simulink model "IEEE34_PMSG"  (R2024a)
settings: Solver=FixedStepDiscrete  StartTime=0.0  StopTime=ttotal  RelTol=1e-3
values from neighbouring files (symbols this model uses):
  C0_300 = 4.9597e-09    [Data_input_DFIG.mat]    (also in Data_input_PMSG.mat)
  C0_301 = 4.8339e-09    [Data_input_DFIG.mat]    (also in Data_input_PMSG.mat)
  C1_300 = 1.0146e-08    [Data_input_DFIG.mat]    (also in Data_input_PMSG.mat)
  C1_301 = 9.7319e-09    [Data_input_DFIG.mat]    (also in Data_input_PMSG.mat)
  CC = [20000 9000 135000 20000 150000 10000 16000 7000 105000 16000 75000 5000 ... (36 elements, 6x6)]    [Data_input_DFIG.mat]    (also in Data_input_PMSG.mat)
  CD = [0 0 34000 135000 0 0 0 7000 0 7000 2000 4000 ... (114 elements, 19x6)]    [Data_input_DFIG.mat]    (also in Data_input_PMSG.mat)
  cte = 1e-06    [Data_input_DFIG.mat]    (also in Data_input_PMSG.mat)
  L0_300 = 0.0039    [Data_input_DFIG.mat]    (also in Data_input_PMSG.mat)
  L0_301 = 0.0043    [Data_input_DFIG.mat]    (also in Data_input_PMSG.mat)
  L1_300 = 0.0014    [Data_input_DFIG.mat]    (also in Data_input_PMSG.mat)
  L1_301 = 0.0014    [Data_input_DFIG.mat]    (also in Data_input_PMSG.mat)
  R0_300 = 1.0909    [Data_input_DFIG.mat]    (also in Data_input_PMSG.mat)
  R0_301 = 1.4885    [Data_input_DFIG.mat]    (also in Data_input_PMSG.mat)
  R1_300 = 0.6983    [Data_input_DFIG.mat]    (also in Data_input_PMSG.mat)
  R1_301 = 1.0537    [Data_input_DFIG.mat]    (also in Data_input_PMSG.mat)
  tf_AB = 1.75    [Data_input_DFIG.mat]    (also in Data_input_PMSG.mat = 2.65)
  tf_ABC = 1.75    [Data_input_DFIG.mat]    (also in Data_input_PMSG.mat = 2.65)
  tf_ABT = 1.75    [Data_input_DFIG.mat]    (also in Data_input_PMSG.mat = 2.65)
  tf_AT = 1.75    [Data_input_DFIG.mat]    (also in Data_input_PMSG.mat = 2.65)
  tf_BC = 1.75    [Data_input_DFIG.mat]    (also in Data_input_PMSG.mat = 2.65)
  tf_BCT = 1.75    [Data_input_DFIG.mat]    (also in Data_input_PMSG.mat = 2.65)
  tf_BT = 1.75    [Data_input_DFIG.mat]    (also in Data_input_PMSG.mat = 2.65)
  tf_CA = 1.75    [Data_input_DFIG.mat]    (also in Data_input_PMSG.mat = 2.65)
  tf_CAT = 1.75    [Data_input_DFIG.mat]    (also in Data_input_PMSG.mat = 2.65)
  tf_CT = 1.75    [Data_input_DFIG.mat]    (also in Data_input_PMSG.mat = 2.65)
  Ts = 5.008e-06    [Data_input_DFIG.mat]    (also in Data_input_PMSG.mat = 1.0016e-05)
undefined symbols (not defined in the file or in its folder): D1, Delta, DiscIntNeverNeededParam, find_system
libraries: spsThreePhaseSeriesRLCLoadLib x31, spsThreePhasePISectionLineLib x22, spsGroundLib x15, spsSeriesRLCLoadLib x14, spsThreePhaseFaultLib x10, spsSecondOrderFilterLib x9, spsPiSectionLineLib x8, spsThreePhaseVIMeasurementLib x6, spsabctodq0Lib x5, simulink_extras x4, spsFirstOrderFilterLib x4, spsThreePhaseTransformerTwoWindingsLib x3
(part 4 of 4)

== system IEEE34_PMSG/Wind Turbine Type 4/Control/Measurement and Transformation/Discrete 3-phase PLL-Driven Positive-Sequence Active & Reactive Power/Discrete 3-phase PLL-Driven Positive-Sequence Fundamental Value/Discrete Variable Frequency Mean value2/Correction subsystem ==
  N : Inport
  F : Inport  Port=2
  In : Inport  Port=3
  Gain1 : Gain  Gain=0.5  SaturateOnIntegerOverflow=on  OutDataTypeStr=Inherit: Same as input  ParamDataTypeStr=Inherit: Same as input
  Product2 : Product  Inputs=*/  InputSameDT=on  SaturateOnIntegerOverflow=on  OutDataTypeStr=Inherit: Same as first input
  Product4 : Product  Inputs=**  InputSameDT=on  SaturateOnIntegerOverflow=on  OutDataTypeStr=Inherit: Same as first input
  Product5 : Product  Inputs=**  InputSameDT=on  SaturateOnIntegerOverflow=on  OutDataTypeStr=Inherit: Same as first input
  Sum1 : Sum  Inputs=+-  InputSameDT=on  SaturateOnIntegerOverflow=on  OutDataTypeStr=Inherit: Same as first input
  Sum4 : Sum  InputSameDT=on  SaturateOnIntegerOverflow=on  OutDataTypeStr=Inherit: Same as first input
  Sum5 : Sum  Inputs=+-  InputSameDT=on  SaturateOnIntegerOverflow=on  OutDataTypeStr=Inherit: Same as first input
  Unit Delay : UnitDelay  SampleTime=Ts  HasFrameUpgradeWarning=on
  Out : Outport  VectorParamsAs1DForOutWhenUnconnected=off
  wires:
  Product4/1 -> Out/1
  Sum4/1 -> Product4/2
  Gain1/1 -> Sum4/1
  Product5/1 -> Gain1/1
  Sum1/1 -> Product5/2
  In/1 -> Sum4/2, Unit Delay/1, Sum1/1
  Product2/1 -> Product4/1
  Sum5/1 -> Product5/1, Product2/1
  F/1 -> Sum5/2
  N/1 -> Product2/2, Sum5/1
  Unit Delay/1 -> Sum1/2

== system IEEE34_PMSG/Wind Turbine Type 4/Control/Measurement and Transformation/Discrete 3-phase PLL-Driven Positive-Sequence Active & Reactive Power/Discrete 3-phase PLL-Driven Positive-Sequence Fundamental Value/Discrete Variable Frequency Mean value2/Discrete Variable Transport Delay ==
  In : Inport
  D : Inport  Port=2
  "S-Function " : S-Function  FunctionName=discreteVariableTransportDelay  Parameters=MaxDelay,Ts,InitialValue  SFunctionDeploymentMode=off  EnableBusSupport=off
  Out : Outport  VectorParamsAs1DForOutWhenUnconnected=off
  wires:
  D/1 -> "S-Function "/2
  In/1 -> "S-Function "/1
  "S-Function "/1 -> Out/1

== system IEEE34_PMSG/Wind Turbine Type 4/Control/Measurement and Transformation/Discrete 3-phase PLL-Driven Positive-Sequence Active & Reactive Power/Discrete 3-phase PLL-Driven Positive-Sequence Fundamental Value2/Discrete Variable Frequency Mean value1/Correction subsystem ==
  N : Inport
  F : Inport  Port=2
  In : Inport  Port=3
  Gain1 : Gain  Gain=0.5  SaturateOnIntegerOverflow=on  OutDataTypeStr=Inherit: Same as input  ParamDataTypeStr=Inherit: Same as input
  Product2 : Product  Inputs=*/  InputSameDT=on  SaturateOnIntegerOverflow=on  OutDataTypeStr=Inherit: Same as first input
  Product4 : Product  Inputs=**  InputSameDT=on  SaturateOnIntegerOverflow=on  OutDataTypeStr=Inherit: Same as first input
  Product5 : Product  Inputs=**  InputSameDT=on  SaturateOnIntegerOverflow=on  OutDataTypeStr=Inherit: Same as first input
  Sum1 : Sum  Inputs=+-  InputSameDT=on  SaturateOnIntegerOverflow=on  OutDataTypeStr=Inherit: Same as first input
  Sum4 : Sum  InputSameDT=on  SaturateOnIntegerOverflow=on  OutDataTypeStr=Inherit: Same as first input
  Sum5 : Sum  Inputs=+-  InputSameDT=on  SaturateOnIntegerOverflow=on  OutDataTypeStr=Inherit: Same as first input
  Unit Delay : UnitDelay  SampleTime=Ts  HasFrameUpgradeWarning=on
  Out : Outport  VectorParamsAs1DForOutWhenUnconnected=off
  wires:
  Product4/1 -> Out/1
  Sum4/1 -> Product4/2
  Gain1/1 -> Sum4/1
  Product5/1 -> Gain1/1
  Sum1/1 -> Product5/2
  In/1 -> Sum4/2, Unit Delay/1, Sum1/1
  Product2/1 -> Product4/1
  Sum5/1 -> Product5/1, Product2/1
  F/1 -> Sum5/2
  N/1 -> Product2/2, Sum5/1
  Unit Delay/1 -> Sum1/2

== system IEEE34_PMSG/Wind Turbine Type 4/Control/Measurement and Transformation/Discrete 3-phase PLL-Driven Positive-Sequence Active & Reactive Power/Discrete 3-phase PLL-Driven Positive-Sequence Fundamental Value2/Discrete Variable Frequency Mean value1/Discrete Variable Transport Delay ==
  In : Inport
  D : Inport  Port=2
  "S-Function " : S-Function  FunctionName=discreteVariableTransportDelay  Parameters=MaxDelay,Ts,InitialValue  SFunctionDeploymentMode=off  EnableBusSupport=off
  Out : Outport  VectorParamsAs1DForOutWhenUnconnected=off
  wires:
  D/1 -> "S-Function "/2
  In/1 -> "S-Function "/1
  "S-Function "/1 -> Out/1

== system IEEE34_PMSG/Wind Turbine Type 4/Control/Measurement and Transformation/Discrete 3-phase PLL-Driven Positive-Sequence Active & Reactive Power/Discrete 3-phase PLL-Driven Positive-Sequence Fundamental Value2/Discrete Variable Frequency Mean value2/Correction subsystem ==
  N : Inport
  F : Inport  Port=2
  In : Inport  Port=3
  Gain1 : Gain  Gain=0.5  SaturateOnIntegerOverflow=on  OutDataTypeStr=Inherit: Same as input  ParamDataTypeStr=Inherit: Same as input
  Product2 : Product  Inputs=*/  InputSameDT=on  SaturateOnIntegerOverflow=on  OutDataTypeStr=Inherit: Same as first input
  Product4 : Product  Inputs=**  InputSameDT=on  SaturateOnIntegerOverflow=on  OutDataTypeStr=Inherit: Same as first input
  Product5 : Product  Inputs=**  InputSameDT=on  SaturateOnIntegerOverflow=on  OutDataTypeStr=Inherit: Same as first input
  Sum1 : Sum  Inputs=+-  InputSameDT=on  SaturateOnIntegerOverflow=on  OutDataTypeStr=Inherit: Same as first input
  Sum4 : Sum  InputSameDT=on  SaturateOnIntegerOverflow=on  OutDataTypeStr=Inherit: Same as first input
  Sum5 : Sum  Inputs=+-  InputSameDT=on  SaturateOnIntegerOverflow=on  OutDataTypeStr=Inherit: Same as first input
  Unit Delay : UnitDelay  SampleTime=Ts  HasFrameUpgradeWarning=on
  Out : Outport  VectorParamsAs1DForOutWhenUnconnected=off
  wires:
  Unit Delay/1 -> Sum1/2
  N/1 -> Sum5/1, Product2/2
  F/1 -> Sum5/2
  Sum5/1 -> Product2/1, Product5/1
  Product2/1 -> Product4/1
  In/1 -> Sum1/1, Unit Delay/1, Sum4/2
  Sum1/1 -> Product5/2
  Product5/1 -> Gain1/1
  Gain1/1 -> Sum4/1
  Sum4/1 -> Product4/2
  Product4/1 -> Out/1

== system IEEE34_PMSG/Wind Turbine Type 4/Control/Measurement and Transformation/Discrete 3-phase PLL-Driven Positive-Sequence Active & Reactive Power/Discrete 3-phase PLL-Driven Positive-Sequence Fundamental Value2/Discrete Variable Frequency Mean value2/Discrete Variable Transport Delay ==
  In : Inport
  D : Inport  Port=2
  "S-Function " : S-Function  FunctionName=discreteVariableTransportDelay  Parameters=MaxDelay,Ts,InitialValue  SFunctionDeploymentMode=off  EnableBusSupport=off
  Out : Outport  VectorParamsAs1DForOutWhenUnconnected=off
  wires:
  "S-Function "/1 -> Out/1
  In/1 -> "S-Function "/1
  D/1 -> "S-Function "/2
